simulink model "polynomial_System"  (R2024a)
settings: Solver=FixedStepDiscrete  StartTime=0.0  StopTime=15  FixedStep=0.25  RelTol=1e-3
values from neighbouring files (symbols this model uses):
  COEFF_A = 1.0    [polynomial_System.sldd]
  COEFF_B = -4.0    [polynomial_System.sldd]
  COEFF_C = 21.0    [polynomial_System.sldd]
settings Model: DataDictionary=polynomial_System.sldd  Creator=ntyler  LastModifiedBy=ntyler

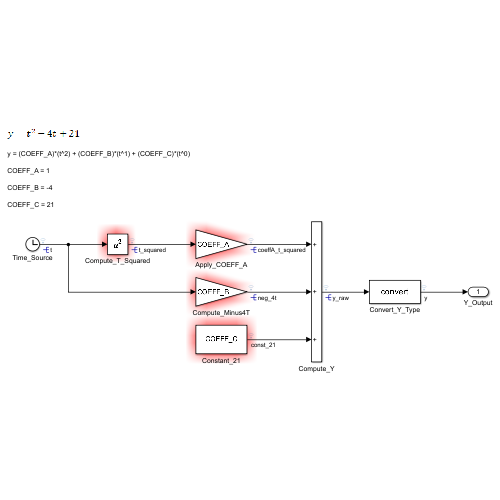
[thumbnail: Simulink's stored preview of the top-level diagram]
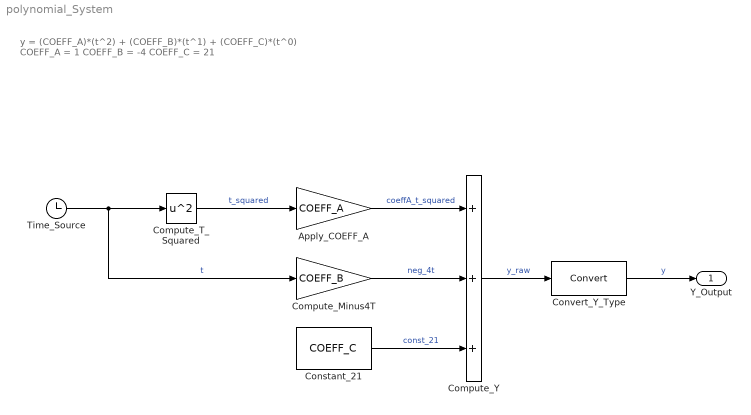
== system polynomial_System ==
  note: y = (COEFF_A)*(t^2) + (COEFF_B)*(t^1) + (COEFF_C)*(t^0)
      | COEFF_A = 1
      | COEFF_B = -4
      | COEFF_C = 21
  Apply_COEFF_A : Gain  Gain=COEFF_A
  Compute_Minus4T : Gain  Gain=COEFF_B
  Compute_T_Squared : Math  Operator=square
  Compute_Y : Sum  Inputs=+++
  Constant_21 : Constant  Value=COEFF_C
  Convert_Y_Type : DataTypeConversion  SaturateOnIntegerOverflow=off  RndMeth=Floor
  Time_Source : Clock
  Y_Output : Outport
  wires:
  Time_Source/1 -> Compute_T_Squared/1, Compute_Minus4T/1  "t"
  Compute_T_Squared/1 -> Apply_COEFF_A/1  "t_squared"
  Apply_COEFF_A/1 -> Compute_Y/1  "coeffA_t_squared"
  Compute_Minus4T/1 -> Compute_Y/2  "neg_4t"
  Constant_21/1 -> Compute_Y/3  "const_21"
  Compute_Y/1 -> Convert_Y_Type/1  "y_raw"
  Convert_Y_Type/1 -> Y_Output/1  "y"
